simulink model "Kalman_EMPhase_noC"  (R2019b)
settings: Solver=VariableStepAuto  StartTime=0.0  StopTime=model.sim_dur  RelTol=1e-3
undefined symbols (not defined in the file or in its folder): Discrete, model, Time
libraries: dspsrcs4 x11, ctrlSharedLib x2
settings Model: Creator=isidoraradenkovic  LastModifiedBy=isidoraradenkovic

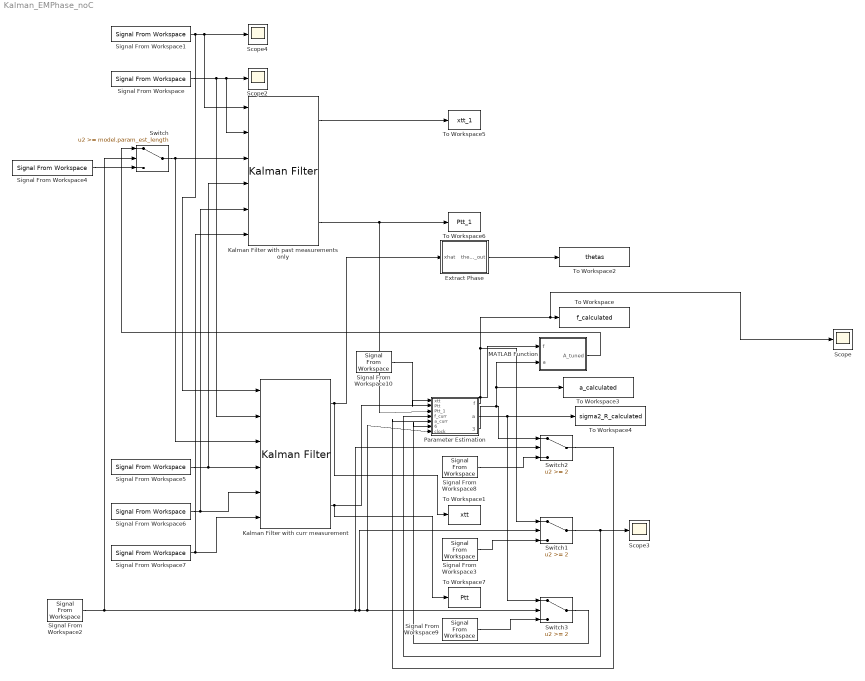
== system Kalman_EMPhase_noC ==
  Extract Phase : MATLAB Function  TreatAsAtomicUnit=on  SystemSampleTime=model.Ts
  Kalman Filter with curr measurement : ctrlSharedLib/Kalman Filter  TimeDomain=Discrete-Time  UseCurrentEstimator=on  ModelSource=Input port  ModelSourceVariable=ss(0.95,1,1,0,1)  A=model.A  B=model.B  C=model.C  D=0  NumberOfStates=2  NumberOfInputs=1  NumberOfOutputs=1  InitialEstimateSource=Dialog  X0=model.x_0  P0=model.Q_const  UseK=off  UseGH=on  NumberOfProcessNoiseInputs=1  G=model.Gm  TimeInvariantG=on  H=0  TimeInvariantH=on  Q=model.Q  TimeInvariantQ=on  R=model.R  TimeInvariantR=on  N=0  TimeInvariantN=on  AddInputPort=on  AddEnablePort=off  OutputEstimatedY=on  OutputP=on  Ts=model.Ts
      settings: SourceProductBaseCode=CT
  Kalman Filter with past measurements only : ctrlSharedLib/Kalman Filter  TimeDomain=Discrete-Time  UseCurrentEstimator=off  ModelSource=Input port  ModelSourceVariable=ss(0.95,1,1,0,1)  A=model.A  B=model.B  C=model.C  D=0  NumberOfStates=2  NumberOfInputs=1  NumberOfOutputs=1  InitialEstimateSource=Dialog  X0=model.x_0  P0=model.Q_const  UseK=off  UseGH=on  NumberOfProcessNoiseInputs=1  G=model.Gm  TimeInvariantG=on  H=0  TimeInvariantH=on  Q=model.Q  TimeInvariantQ=on  R=model.R  TimeInvariantR=on  N=0  TimeInvariantN=on  AddInputPort=on  AddEnablePort=off  OutputEstimatedY=on  OutputP=on  Ts=model.Ts
      settings: SourceProductBaseCode=CT
  MATLAB Function : MATLAB Function  TreatAsAtomicUnit=on  SystemSampleTime=model.Ts
  Parameter Estimation : MATLAB Function  TreatAsAtomicUnit=on  SystemSampleTime=model.Ts
  Scope{,2..4} (4 alike) : Scope
  Signal From Workspace : dspsrcs4/Signal From Workspace  X=input_data  Ts=model.Ts  nsamps=1  OutputAfterFinalValue=Cyclic repetition  ignoreOrWarnInputAndFrameLengths=off  OutputFrames=off
  Signal From Workspace1 : dspsrcs4/Signal From Workspace  X=tms_pulses  Ts=model.Ts  nsamps=1  OutputAfterFinalValue=Cyclic repetition  ignoreOrWarnInputAndFrameLengths=off  OutputFrames=off
  Signal From Workspace10 : dspsrcs4/Signal From Workspace  X=out.xtt  Ts=model.Ts  nsamps=1  OutputAfterFinalValue=Cyclic repetition  ignoreOrWarnInputAndFrameLengths=off  OutputFrames=off
  Signal From Workspace2 : dspsrcs4/Signal From Workspace  X=1:1:(6*model.param_est_length)  Ts=model.Ts  nsamps=1  OutputAfterFinalValue=Holding final value  ignoreOrWarnInputAndFrameLengths=off  OutputFrames=off
  Signal From Workspace3 : dspsrcs4/Signal From Workspace  X=model.f  Ts=model.Ts  nsamps=1  OutputAfterFinalValue=Cyclic repetition  ignoreOrWarnInputAndFrameLengths=off  OutputFrames=off
  Signal From Workspace4 : dspsrcs4/Signal From Workspace  X=model.A  Ts=model.Ts/2  nsamps=2  OutputAfterFinalValue=Cyclic repetition  ignoreOrWarnInputAndFrameLengths=off  OutputFrames=off
  Signal From Workspace5 : dspsrcs4/Signal From Workspace  X=model.B  Ts=model.Ts/2  nsamps=2  OutputAfterFinalValue=Cyclic repetition  ignoreOrWarnInputAndFrameLengths=off  OutputFrames=off
  Signal From Workspace6 : dspsrcs4/Signal From Workspace  X=model.C  Ts=model.Ts  nsamps=1  OutputAfterFinalValue=Cyclic repetition  ignoreOrWarnInputAndFrameLengths=off  OutputFrames=off
  Signal From Workspace7 : dspsrcs4/Signal From Workspace  X=model.D  Ts=model.Ts  nsamps=1  OutputAfterFinalValue=Cyclic repetition  ignoreOrWarnInputAndFrameLengths=off  OutputFrames=off
  Signal From Workspace8 : dspsrcs4/Signal From Workspace  X=model.a  Ts=model.Ts/2  nsamps=2  OutputAfterFinalValue=Cyclic repetition  ignoreOrWarnInputAndFrameLengths=off  OutputFrames=off
  Signal From Workspace9 : dspsrcs4/Signal From Workspace  X=model.sigma2_R  Ts=model.Ts  nsamps=1  OutputAfterFinalValue=Cyclic repetition  ignoreOrWarnInputAndFrameLengths=off  OutputFrames=off
  Switch : Switch  Threshold=model.param_est_length
  Switch1 : Switch  Threshold=2
  Switch2 : Switch  Threshold=2
  Switch3 : Switch  Threshold=2
  To Workspace : ToWorkspace  VariableName=f_calculated  SampleTime=model.Ts
      settings: MaxDataPoints=1  Save2DSignal=2-D array (concatenate along first dimension)
  To Workspace1 : ToWorkspace  VariableName=xtt  SampleTime=model.Ts
      settings: Save2DSignal=2-D array (concatenate along first dimension)
  To Workspace2 : ToWorkspace  VariableName=thetas  SampleTime=model.Ts
      settings: Save2DSignal=2-D array (concatenate along first dimension)
  To Workspace3 : ToWorkspace  VariableName=a_calculated  SampleTime=model.Ts
      settings: MaxDataPoints=2  Save2DSignal=2-D array (concatenate along first dimension)
  To Workspace4 : ToWorkspace  VariableName=sigma2_R_calculated  SampleTime=model.Ts
      settings: MaxDataPoints=1  Save2DSignal=2-D array (concatenate along first dimension)
  To Workspace5 : ToWorkspace  VariableName=xtt_1  SampleTime=model.Ts
      settings: Save2DSignal=2-D array (concatenate along first dimension)
  To Workspace6 : ToWorkspace  VariableName=Ptt_1  SampleTime=model.Ts
      settings: Save2DSignal=2-D array (concatenate along first dimension)
  To Workspace7 : ToWorkspace  VariableName=Ptt  SampleTime=model.Ts
      settings: Save2DSignal=2-D array (concatenate along first dimension)
  wires:
  Kalman Filter with past measurements only/3 -> Parameter Estimation/3(Ptt_1), To Workspace6/1
  Signal From Workspace5/1 -> Kalman Filter with curr measurement/4, Kalman Filter with past measurements only/4
  Signal From Workspace6/1 -> Kalman Filter with curr measurement/5, Kalman Filter with past measurements only/5
  Parameter Estimation/3(sigmaR) -> Switch3/1, To Workspace4/1
  Switch/1 -> Kalman Filter with past measurements only/3, Kalman Filter with curr measurement/3
  Signal From Workspace/1 -> Scope2/1, Kalman Filter with past measurements only/2, Kalman Filter with curr measurement/2
  Parameter Estimation/1(f) -> MATLAB Function/1(f), Scope/1, To Workspace/1, Switch1/1
  Signal From Workspace2/1 -> Switch2/2, Parameter Estimation/7(clock), Switch3/2, Switch1/2, Switch/2
  Parameter Estimation/2(a) -> MATLAB Function/2(a), To Workspace3/1, Switch2/1
  Signal From Workspace1/1 -> Scope4/1, Kalman Filter with past measurements only/1, Kalman Filter with curr measurement/1
  Extract Phase/1(thetas_out) -> To Workspace2/1
  Kalman Filter with past measurements only/1 -> To Workspace5/1
  Signal From Workspace4/1 -> Switch/3
  MATLAB Function/1(A_tuned) -> Switch/1
  Switch1/1 -> Scope3/1, Parameter Estimation/4(f_curr)
  Signal From Workspace9/1 -> Switch3/3
  Kalman Filter with curr measurement/3 -> Parameter Estimation/2(Ptt), To Workspace7/1
  Signal From Workspace8/1 -> Switch2/3
  Switch2/1 -> Parameter Estimation/5(a_curr)
  Signal From Workspace7/1 -> Kalman Filter with curr measurement/6, Kalman Filter with past measurements only/6
  Switch3/1 -> Parameter Estimation/6(sigmaR_curr)
  Signal From Workspace3/1 -> Switch1/3
  Kalman Filter with curr measurement/1 -> Extract Phase/1(xhat), To Workspace1/1
  Signal From Workspace10/1 -> Parameter Estimation/1(xtt)

== matlab function Kalman_EMPhase_noC/Parameter Estimation ==
  settings: sampleTime=1
  data: xtt input; Ptt input; f output size=model.num_rhythms; Ptt_1 input; a output size=[2*model.num_rhythms, 2*model.num_rhythms]; sigmaR output size=model.num_rhythms; model parameter; f_curr input; a_curr input; sigmaR_curr input; clock input
function [f, a, sigmaR]  = parameter_estimation(xtt, Ptt, Ptt_1, model, f_curr, a_curr, sigmaR_curr, clock)

%WARNING!!!!!! To-do: add dimensions_param = model.state_dimensions;
%Right now, 2 is used as a dimension because Simulink complains when
%variables are used for matrix dimensions. When the state space is
%extended for artefact removal, change the 2's to a new value.
%Warning No2: note the limits imposed on model parameters, such as how
%many samples we use to do EM. If this starts causing errors, ensure
%that you are using last n samples where n is at most the max used here.
%model = model;

if clock == model.param_est_length+1
    %%Backward Smoothing
    [PttN, xttN, Ptt_1N, xforwN, PforwN] = backward_smoothing(model, Ptt, Ptt_1, xtt);
    
    %%EM parameter estimation
    [f, a, sigmaR]  = em_method(model, PttN, xttN, Ptt_1N, xforwN, PforwN);
    %     f = f_value(1);
    %     a = a_value(1:2, 1:2);
    %     sigmaR = sigmaR_value(1);
else
    f = f_curr;
    a = a_curr;
    sigmaR = sigmaR_curr;
end

    function [PttN, xttN, Ptt_1N, xforwN, PforwN] = backward_smoothing(model, Ptt, Ptt_1, xtt)
        length_param = model.param_est_length; %Limit to a max of 5000, BUT product limit is 10000
        
        PttN = zeros(min(2 * length_param, 10000), 2); % For the smoothing step
        xttN = zeros(min(length_param, 5000), 2);
        Ptt_1N = zeros(min(2 * length_param, 10000), 2); % Covariance
        
        coder.varsize('xforwN');
        coder.varsize('PforwN');
        xforwN = xtt(length_param+1, :);
        PforwN = Ptt((2 * length_param+1):(2 * (length_param+1)), :);
        
        
        for j= (length_param+1):(-1):2 % The paper is 0 indexed, MATLAB is 1 indexed
            % Extract matrices for simpler representation
            % Index (j-1) becomes:
            % ((j-2)*dimensions_param+1):((j-1)*dimensions_param)
            % Index j becomes:
            % ((j-1)*dimensions_param+1):(j*dimensions_param)
            
            ind_prev = max((j-2)*2+1, 1):min((j-1)*2, 50000);
            ind_curr = max((j-1)*2+1, 1):min(j*2, 50000);
            
            Pt_1_prev = Ptt_1(ind_prev, :);
            Pt_1_curr = Ptt_1(ind_curr, :);
            Pt_prev = Ptt(ind_prev, :);
            %xt_prev = xtt(j-1, :);
            xt_prev = xtt(j-1, 1:2);
            
            J = Pt_1_prev\Pt_prev*model.A'; %UNSTABLE INVERSES?
            xttN(j-1, min(1:2, 10:11)) = xt_prev+(xforwN-xt_prev*(model.A'))*(J');
            PttN(ind_prev, min(1:2, 10:11)) = Pt_prev+J*(PforwN-Pt_1_curr)*J';
            %covariance is symmetric, so Ptt_1N = Pt_1tN = J*PttN hence:
            Ptt_1N(ind_prev, min(1:2, 10:11)) = J*PforwN;
            
            xforwN = xttN(j-1, :);
            PforwN = PttN(ind_prev, :);
        end
        
    end

    function [f, a, sigmaR]  = em_method(model, PttN, xttN, Ptt_1N, xforwN, PforwN)
        length_param = model.param_est_length;
        num_rhythms = model.num_rhythms;
        
        P_A = matrix_sum(PttN, 2);
        P_B = matrix_sum(Ptt_1N, 2);
        P_C = matrix_sum([PttN((2+1):end, :); PforwN], 2);
        
        xtN = [xttN(2:min(length_param, 5000), :); xforwN];
        x_A_prod = matrix_product(xttN, xttN, 2);
        x_A = matrix_sum(x_A_prod, 2);
        x_B_prod = matrix_product(xtN, xttN, 2);
        x_B = matrix_sum(x_B_prod, 2);
        x_C_prod = matrix_product(xtN, xtN, 2);
        x_C = matrix_sum(x_C_prod, 2);
        
        A_smooth = P_A+x_A;
        B_smooth = P_B+x_B;
        C_smooth = P_C+x_C;
        
        f_temp = atan(rt(B_smooth, num_rhythms)./tr(B_smooth, num_rhythms));
        a_temp = sqrt(rt(B_smooth, num_rhythms).^2+tr(B_smooth, num_rhythms).^2)./tr(A_smooth, num_rhythms);
        sigmaR_temp = double(tr(C_smooth, num_rhythms)-(a_temp.^2).*tr(A_smooth, num_rhythms))./double(2*length_param);
        
        f = mod(f_temp(1)+2, 2)*pi;
        a = a_temp(1)*eye(2);
        sigmaR = sigmaR_temp(1);
    end

end

== matlab function Kalman_EMPhase_noC/Extract Phase ==
  data: xhat input; thetas_out output
function thetas_out  = extract_phase(xhat)
num_rhythms = length(xhat)/2;
% thetas_out = zeros(num_rhythms, 1);
% 
% for j = 1:num_rhythms
%     Im = xhat(2 * (j-1) + 2);
%     Re = xhat(2 * (j-1) + 1);
%     thetas_out(j, 1) = atan2(Im, Re);
% end

thetas_out = atan2(xhat(2:2:2*num_rhythms), xhat(1:2:2*(num_rhythms-1)+1))

== matlab function Kalman_EMPhase_noC/MATLAB Function ==
  data: A_tuned output; f input; a input; model parameter
function A_tuned = tune_A(f, a, model)
angles = 2*pi*model.Ts*f;
rot_cell = cell(1); % GENERALISE FOR MULTIPLE FREQ TRACKING

for j = 1:1 % model.num_rhythms GENERALISE FOR MULTIPLE FREQ TRACKING
    rot_j = [cos(angles(j)) -sin(angles(j)); sin(angles(j)) cos(angles(j))];
    rot_cell{j} = rot_j;
end
rot =blkdiag(rot_cell{1}); % GENERALISE FOR MULTIPLE FREQ TRACKING

A_tuned = a*rot;
